simulink model "GPS_processing_test"  (R2016b)
settings: Solver=VariableStepAuto  StartTime=0.0  StopTime=60  RelTol=1e-3
values from neighbouring files (symbols this model uses):
  fsw_params = init_fsw_params()    [GPS_processing_test_init.m]
libraries: gps x1, GPS_processing_lib x1, GPS_time_lib x1, MET_lib x1, time_coord_rotation_lib x1, tle2eci_coarse_lib x1
settings Model: Creator=Taylor  LastModifiedBy=Taylor

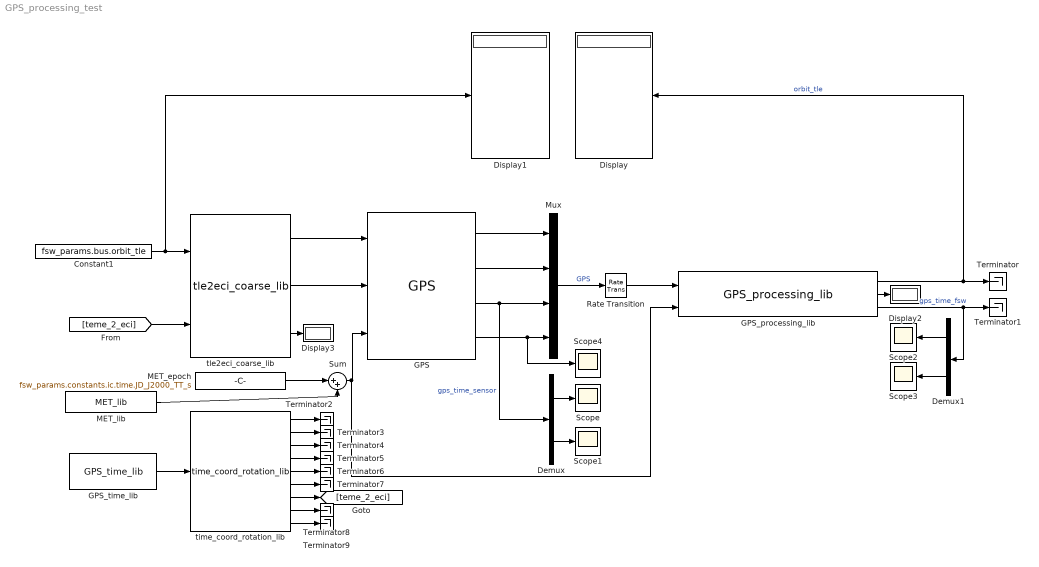
== system GPS_processing_test ==
  Constant1 : Constant  Value=fsw_params.bus.orbit_tle
  Demux : Demux  Outputs=2
  Demux1 : Demux  Outputs=2
  Display{,1..3} (4 alike) : Display
  GPS : gps/GPS
  GPS_processing_lib : GPS_processing_lib/GPS_processing_lib
  GPS_time_lib : GPS_time_lib/GPS_time_lib
  MET_epoch : Constant  Value=fsw_params.constants.ic.time.JD_J2000_TT_s
  MET_lib : MET_lib/MET_lib
  Mux : Mux  Inputs=[3 3 2 1]
  Rate Transition : RateTransition  X0=fsw_params.sensor_processing.gps.ic.all  OutPortSampleTime=fsw_params.sensor_processing.gps.sample_time_s
  Scope{,1..4} (5 alike) : Scope
  Sum : Sum  Inputs=|++
  Terminator{,1..9} (10 alike) : Terminator
  time_coord_rotation_lib : time_coord_rotation_lib/time_coord_rotation_lib
  tle2eci_coarse_lib : tle2eci_coarse_lib/tle2eci_coarse_lib
  wires:
  GPS_processing_lib/1 -> Display/1, Terminator/1  "orbit_tle"
  GPS_processing_lib/3 -> Terminator1/1, Demux1/1  "gps_time_fsw"
  GPS/4 -> Scope4/1, Mux/4
  Mux/1 -> Rate Transition/1  "GPS"
  GPS/3 -> Mux/3, Demux/1  "gps_time_sensor"
  GPS/2 -> Mux/2
  GPS/1 -> Mux/1
  Constant1/1 -> Display1/1, tle2eci_coarse_lib/1
  Demux/1 -> Scope/1
  Demux/2 -> Scope1/1
  tle2eci_coarse_lib/1 -> GPS/1
  tle2eci_coarse_lib/2 -> GPS/2
  Demux1/1 -> Scope2/1
  Demux1/2 -> Scope3/1
  GPS_processing_lib/2 -> Display2/1
  GPS_time_lib/1 -> time_coord_rotation_lib/1
  time_coord_rotation_lib/7 -> [teme_2_eci]
  [teme_2_eci] -> tle2eci_coarse_lib/2
  time_coord_rotation_lib/1 -> Terminator2/1
  time_coord_rotation_lib/2 -> Terminator3/1
  time_coord_rotation_lib/3 -> Terminator4/1
  time_coord_rotation_lib/4 -> Terminator5/1
  time_coord_rotation_lib/5 -> Terminator6/1
  time_coord_rotation_lib/6 -> Terminator7/1
  time_coord_rotation_lib/8 -> Terminator8/1
  time_coord_rotation_lib/9 -> Terminator9/1
  tle2eci_coarse_lib/3 -> Display3/1
  Rate Transition/1 -> GPS_processing_lib/1
  MET_lib/1 -> Sum/2
  MET_epoch/1 -> Sum/1
  Sum/1 -> GPS_processing_lib/2, GPS/3
